simulink model "Excercise_1"  (R2021b)
settings: Solver=ode4  StartTime=0.0  StopTime=50  FixedStep=0.05  RelTol=1e-3
values from neighbouring files (symbols this model uses):
  ActiveMode =     [AC_System_Variables.mat]
  command =     [AC_System_Variables.mat]
  RequestedMode =     [AC_System_Variables.mat]
  state =     [AC_System_Variables.mat]
undefined symbols (not defined in the file or in its folder): sigbuilder_block
settings Model: Creator=t  LastModifiedBy=t

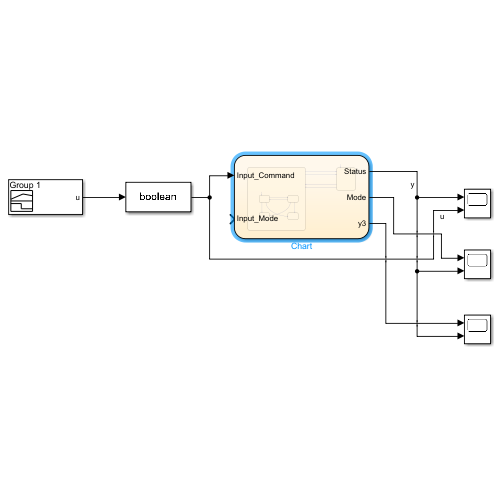
[thumbnail: Simulink's stored preview of the top-level diagram]
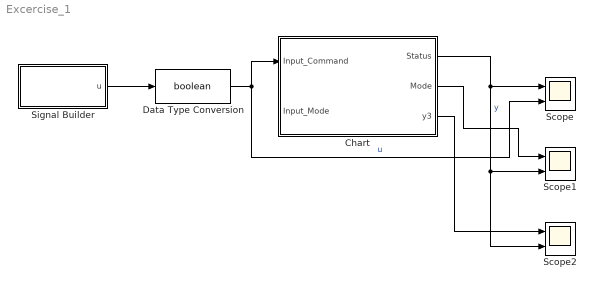
== system Excercise_1 ==
  Chart : Stateflow chart  TreatAsAtomicUnit=on
  Data Type Conversion : DataTypeConversion  OutDataTypeStr=boolean
  Scope : Scope  NumInputPorts=2
  Scope1 : Scope  NumInputPorts=2
  Scope2 : Scope  NumInputPorts=2
  Signal Builder : Subsystem  Tag=STV Subsys  LoadFcn=sigbuilder_block('load');  StartFcn=sigbuilder_block('start');  StopFcn=sigbuilder_block('stop');  ClipboardFcn=sigbuilder_block('clipboard');  mask(Sigbuilder block){tuvar=[0:10]}
      mask help: Simulink:masks:SigbuilderBlock_MD
      mask init:
      | if ~strcmp(get_param(bdroot(gcbh),'SimulationStatus'),'stopped') tuvar = sigbuilder_block('maskInit'); end
      settings: CopyFcn=sigbuilder_block('copy');  DeleteFcn=sigbuilder_block('delete');  ModelCloseFcn=sigbuilder_block('modelClose');  PreSaveFcn=sigbuilder_block('preSave');  PauseFcn=sigbuilder_block('pause');  ContinueFcn=sigbuilder_block('continue');  NameChangeFcn=sigbuilder_block('namechange');  OpenFcn=sigbuilder_block('open',[0 30 1152 561.6 ]);  CloseFcn=sigbuilder_block('close');
      mask Display: plot(0, 0, 100, 100,[2, 2, 32, 32, 2], [68, 8, 8, 68, 68],[32, 2], [38, 38], [32, 19, 2],[53, 60, 44], [32, 17, 17, 2],[16, 16, 31, 31]);txt = getActiveGroup(gcbh);text(2, 100, txt,'verticalAlignment', 'top');
  wires:
  Signal Builder/1(u) -> Data Type Conversion/1
  Data Type Conversion/1 -> Scope/2, Chart/1(Input_Command)  "u"
  Chart/1(Status) -> Scope/1, Scope1/2, Scope2/2  "y"
  Chart/2(Mode) -> Scope1/1
  Chart/3(y3) -> Scope2/1

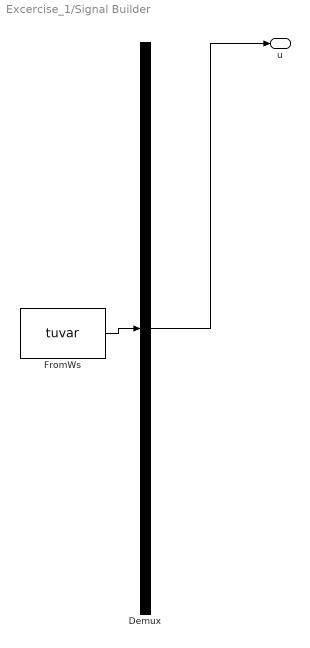
== system Excercise_1/Signal Builder ==
  Demux : Demux  Tag=STV Demux  Outputs=1
      settings: DisplayOption=none
  FromWs : FromWorkspace  Tag=STV FromWs  VariableName=tuvar
      SigBuilderData=|
      | common.afterFinalStr = 'Extrapolate'
      | common.sampleTime = 0
      | dataSet.timeRange = [0 50]
      | dataSet.name = 'Group 1'
      | sbobj.Groups.Name = 'Group 1'
      | sbobj.Groups.Signals.Name = 'u'
      | sbobj.Groups.Signals.XData = [0 1.3 1.3 16 16 24 24 35 35 40 40 47 47 50]
      | sbobj.Groups.Signals.YData = [0 0 1 1 0 0 1 1 0 0 1 1 0 0]
      | sbobj.Groups.TimeRange = [0 50]
  u : Outport  Tag=STV Outport
  wires:
  Demux/1 -> u/1
  FromWs/1 -> Demux/1

== stateflow chart Excercise_1/Chart ==
  state ON
    entry: y=state.ON
    during: y=state.ON
    during: counter=counter+1
    ex: counter=0
    on before(5,sec):
    y2=y2+3
    on every(50,tick):
    y3=y3+6
    on at(150,tick):
    y3=15
  state OFF
    entry: y=state.OFF
    during: y=state.OFF
    during: counter=counter+1
    ex: counter=0
    on after(3000,tick):
    y2=y2+5
    on every(30,tick):
    y3=y3+1
  (default) -> OFF
  ON -> OFF [order 1] : [u==command.OFF]
  ON -> OFF [order 2] : [after(10,sec)]
  OFF -> ON [order 1] : [u==command.ON]
  OFF -> ON [order 2] : [after(20,sec)]
  data: Input_Command input; Status output; command parameter; state parameter; counter local uint8 =uint8(0); limit constant uint8 =20; Mode output =0; y3 output =0; RequestedMode parameter; ActiveMode parameter; Input_Mode input
